simulink model "MassSpringDamped_Problem"  (R2022a)
settings: Solver=VariableStepAuto  StartTime=0.0  StopTime=10  MaxStep=1e-4  RelTol=1e-3
values from neighbouring files (symbols this model uses):
  c = 4    [msd_params.m]
  k = 400    [msd_params.m]
  m = 1    [msd_params.m]
settings Model: Creator=teacherforward  LastModifiedBy=teacherforward

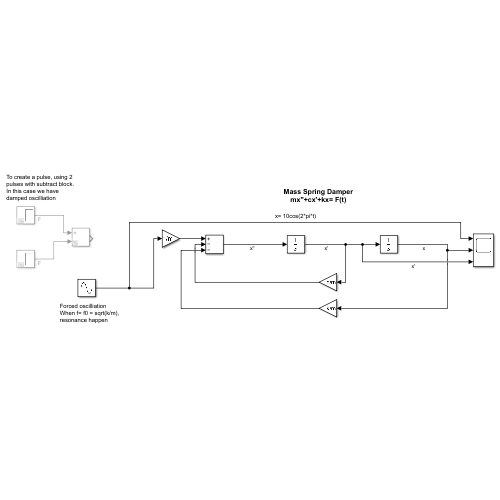
[thumbnail: Simulink's stored preview of the top-level diagram]
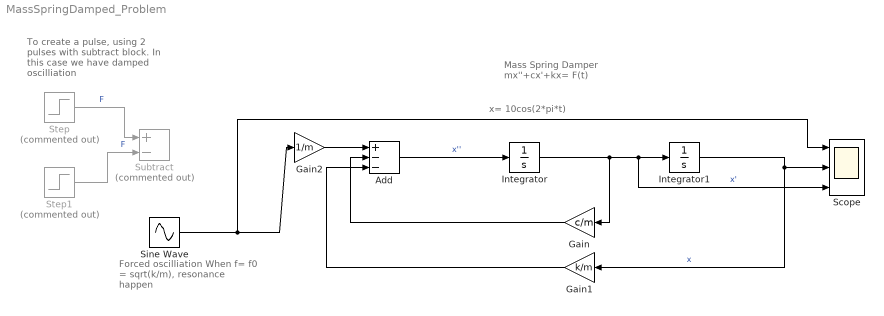
== system MassSpringDamped_Problem ==
  note: Forced oscilliation
      | When f= f0 = sqrt(k/m), resonance happen
  note: x= 10cos(2*pi*t)
  note: To create a pulse, using 2 pulses with subtract block. In this case we have damped oscilliation
  note: Mass Spring Damper
      | mx''+cx'+kx= F(t)
  Add : Sum  Inputs=+--
  Gain : Gain  Gain=c/m
  Gain1 : Gain  Gain=k/m
  Gain2 : Gain  Gain=1/m
  Integrator : Integrator
  Integrator1 : Integrator
  Scope : Scope  NumInputPorts=3
  Sine Wave : Sin  Amplitude=10  Frequency=sqrt(k/m)  SampleTime=0
  Step : Step  Commented=on  Time=2.0  After=20  SampleTime=0
  Step1 : Step  Commented=on  Time=2.1  After=20  SampleTime=0
  Subtract : Sum  Commented=on  Inputs=+-
  wires:
  Integrator/1 -> Gain/1, Scope/3, Integrator1/1  "x'"
  Integrator1/1 -> Gain1/1, Scope/2  "x"
  Add/1 -> Integrator/1  "x''"
  Gain/1 -> Add/2
  Gain1/1 -> Add/3
  Gain2/1 -> Add/1
  Step/1 -> Subtract/1  "F"
  Step1/1 -> Subtract/2  "F"
  Sine Wave/1 -> Scope/1, Gain2/1
